simulink model "builder_system"  (R2024b)
settings: Solver=FixedStepAuto  StartTime=0.0  StopTime=50  RelTol=1e-3
libraries: arduinolib x2, svdutilitieslib x1
settings Model: DataDictionary=data_struct.sldd  ExtModeTrigDuration=2  Creator=Nitesh  LastModifiedBy=Nitesh
settings SolverCC: AutoInsertRateTranBlk=on
settings OptimizationCC: EnhancedBackFolding=on  PassReuseOutputArgsAs=Individual arguments  ZeroExternalMemoryAtStartup=off  ZeroInternalMemoryAtStartup=off  MaxStackSize=64  OptimizeBlockOrder=speed  DifferentSizesBufferReuse=on  OptimizationCustomize=off  EfficientTunableParamExpr=on
settings DebuggingCC: ParameterTunabilityLossMsg=error
settings HardwareCC: ProdBitPerPointer=32  ProdBitPerSizeT=32  ProdBitPerPtrDiffT=32  ProdLargestAtomicInteger=Long  ProdLargestAtomicFloat=Double  ProdWordSize=32  ProdLongLongMode=on  ProdHWDeviceType=ARM Compatible->ARM Cortex  UseEmbeddedCoderFeatures=off
settings SFSimCC: MATLABDynamicMemAlloc=off
settings RTWCC: Description=Embedded Coder  SystemTargetFile=ert.tlc  HardwareBoard=ESP32-WROOM(Arduino Compatible)  TLCOptions="-aInlineSetEventsForThisBaseRateFcn=TLC_FALSE -aSuppressMultiTaskScheduler=TLC_FALSE  -aRateBasedStepFcn=0"  TemplateMakefile=ert_default_tmf  Toolchain=ESP32  BuildConfiguration=Debug
settings CodeAppCC: ForceParamTrailComments=on  IgnoreCustomStorageClasses=off  OperatorAnnotations=on  SimulinkDataObjDesc=on  SFDataObjDesc=on  InsertBlockDesc=on
settings ERTTargetCC: SupportContinuousTime=on  SupportNonInlinedSFcns=on  SupportVariableSizeSignals=on  ExtModeTransport=3  ExtModeStaticAlloc=on  ExtModeAutomaticAllocSize=off  ExtModeStaticAllocSize=65536  ExtModeMexFile=ext_xcp  ExtModeIntrfLevel=Level2 - Open  InlinedParameterPlacement=Hierarchical

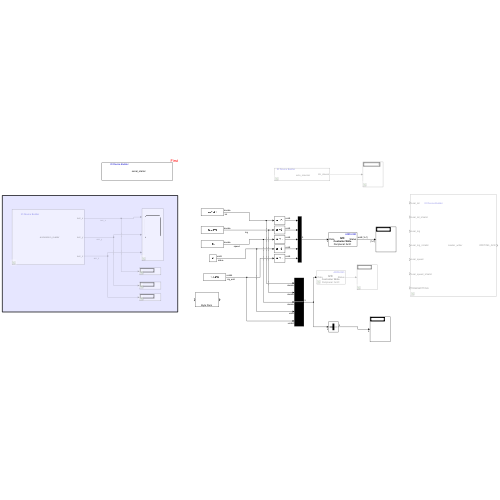
[thumbnail: Simulink's stored preview of the top-level diagram]
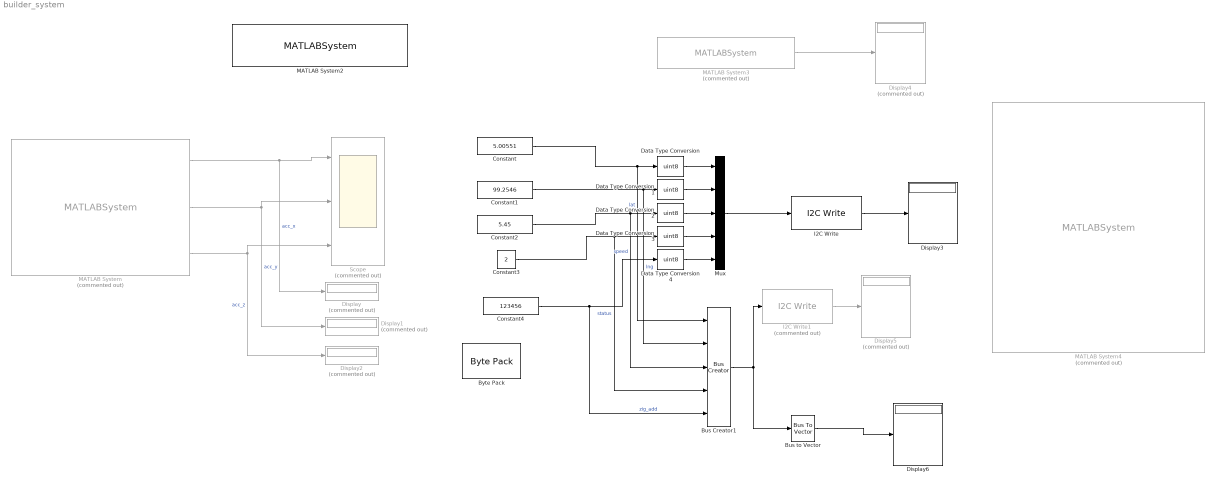
== system builder_system ==
  Bus Creator1 : BusCreator  Inputs=5  OutDataTypeStr=Bus: data_packet
  Bus to Vector : BusToVector
  Byte Pack : svdutilitieslib/Byte Pack  maskPackedDataType=uint8  datatypes={'double'}  byteAlign=1  blockPlatform=arduinoert
  Constant : Constant  Value=5.00551  OutDataTypeStr=double
  Constant1 : Constant  Value=99.2546  OutDataTypeStr=double
  Constant2 : Constant  Value=5.45  OutDataTypeStr=double
  Constant3 : Constant  Value=2  OutDataTypeStr=uint8
  Constant4 : Constant  Value=123456  OutDataTypeStr=uint64
  Data Type Conversion{,1..4} (5 alike) : DataTypeConversion  OutDataTypeStr=uint8  SaturateOnIntegerOverflow=off  RndMeth=Floor
  Display{,1..2,4..5} (5 alike) : Display  Commented=on
  Display3 : Display
  Display6 : Display
  I2C Write : arduinolib/I2C Write  I2CModule=0  Mode=Master  SlaveAddress=60  SlaveByteOrder=BigEndian  Direction=Transmitter  RegisterAddressMode=on  RegisterAddress=0  SlaveDataType=uint8  DataLength=1  NoAck=off  RepeatedStart=off  OutputStatus=on  blockPlatform=ARDUINO
      settings: SourceProductName=Common
  I2C Write1 : arduinolib/I2C Write  Commented=on  I2CModule=0  Mode=Master  SlaveAddress=60  SlaveByteOrder=BigEndian  Direction=Transmitter  RegisterAddressMode=on  RegisterAddress=0  SlaveDataType=uint8  DataLength=1  NoAck=off  RepeatedStart=off  OutputStatus=on  blockPlatform=ARDUINO
      settings: SourceProductName=Common
  MATLAB System : MATLABSystem  Priority=2  Commented=on  System=accleration_reader  ACCEL_RANGE=uint8( 2 )  ENABLE_GYRO=boolean( 0 )  DLPF_SETTING=uint8( 0 )  SampleTime=-1
      mask Type: accleration_reader
      mask Display:
      | color('white');plot([100,100,100,100]*1,[100,100,100,100]*1);plot([100,100,100,100]*0,[100,100,100,100]*0);color('blue');text(38, 92, 'IO Device Builder','horizontalAlignment', 'right');
      | color('black');text(52,50,' accleration_reader','horizontalAlignment','center');
      | port_label('output',1,'acc_x');port_label('output',2,'acc_y');port_label('output',3,'acc_z');
  MATLAB System2 : MATLABSystem  ExecutionOrder=First  System=serial_starter  SampleTime=-1
      mask Type: serial_starter
      mask Display:
      | color('white');plot([100,100,100,100]*1,[100,100,100,100]*1);plot([100,100,100,100]*0,[100,100,100,100]*0);color('blue');text(38, 92, 'IO Device Builder','horizontalAlignment', 'right');
      | color('black');text(52,50,' serial_starter','horizontalAlignment','center');
  MATLAB System3 : MATLABSystem  Priority=1  Commented=on  System=wire_scanner  SampleTime=-1
      mask Type: wire_scanner
      mask Display:
      | color('white');plot([100,100,100,100]*1,[100,100,100,100]*1);plot([100,100,100,100]*0,[100,100,100,100]*0);color('blue');text(38, 92, 'IO Device Builder','horizontalAlignment', 'right');
      | color('black');text(52,50,' wire_scanner','horizontalAlignment','center');
      | port_label('output',1,'i2c_slaves');
  MATLAB System4 : MATLABSystem  Priority=1  Commented=on  System=master_writer  slave_address=uint16( 60 )  bus_frequency=uint64( 100000 )  SampleTime=-1
      mask Type: master_writer
      mask Display:
      | color('white');plot([100,100,100,100]*1,[100,100,100,100]*1);plot([100,100,100,100]*0,[100,100,100,100]*0);color('blue');text(38, 92, 'IO Device Builder','horizontalAlignment', 'right');
      | color('black');text(52,50,' master_writer','horizontalAlignment','center');
      | port_label('input',1,'local_lat');port_label('input',2,'local_lat_isValid');port_label('input',3,'local_lng');port_label('input',4,'local_lng_inValid');port_label('input',5,'local_speed');port_label('input',6,'local_speed_isValid');port_label('input',7,'TRANSMITTING');port_label('output',1,'WRITING_ACK');
  Mux : Mux  Inputs=5
  Scope : Scope  Commented=on  NumInputPorts=3
  wires:
  MATLAB System/1 -> Display/1, Scope/1  "acc_x"
  MATLAB System/2 -> Display1/1, Scope/2  "acc_y"
  MATLAB System/3 -> Display2/1, Scope/3  "acc_z"
  Constant1/1 -> Bus Creator1/2, Data Type Conversion1/1  "lng"
  Constant/1 -> Bus Creator1/1, Data Type Conversion/1  "lat"
  Constant2/1 -> Bus Creator1/3, Data Type Conversion2/1  "speed"
  MATLAB System3/1 -> Display4/1
  Mux/1 -> I2C Write/1
  I2C Write/1 -> Display3/1
  Constant3/1 -> Bus Creator1/4, Data Type Conversion3/1  "status"
  Constant4/1 -> Bus Creator1/5, Data Type Conversion4/1  "zig_add"
  Data Type Conversion/1 -> Mux/1
  Data Type Conversion1/1 -> Mux/2
  Data Type Conversion2/1 -> Mux/3
  Data Type Conversion3/1 -> Mux/4
  Data Type Conversion4/1 -> Mux/5
  I2C Write1/1 -> Display5/1
  Bus Creator1/1 -> Bus to Vector/1, I2C Write1/1
  Bus to Vector/1 -> Display6/1
